simulink model "METI_TRAMI_Thermal_ver01_Jmaab_2018b_Intg"  (R2018b)
settings: Solver=ode8  StartTime=0  StopTime=end_time  FixedStep=sampling_time  RelTol=1e-3
PreLoadFcn:
  | METI_TRAMI_Thermal_ver01_Jmaab_PreLoad;
values from neighbouring files (symbols this model uses):
  degC2K = 273.15    [METI_TRAMI_Thermal_ver01_Jmaab_PreLoad.m]    (also in init_setting_METI.m)
  K2degC = -273.15    [METI_TRAMI_Thermal_ver01_Jmaab_PreLoad.m]    (also in init_setting_METI.m)
undefined symbols (not defined in the file or in its folder): ACC_D_Gain, ACC_I_Gain, ACC_P_Gain, ALT_CNT_ALT_OFF_RPM_HYS_rpm, ALT_CNT_ALT_ON_RPM_HYS_rpm, ALT_CNT_Alter_V_BASE_V, ALT_CNT_Alter_V_Kaisei_V, ALT_CNT_flag_disable_kaisei, ALT_CNT_V_Battely_Kudo_V, ALT_PNT_ALT_GDCurrent_A, ALT_PNT_ALT_GDVolt_V, ALT_PNT_Alter_limit_Current_V_table, ALT_PNT_Alter_limit_Current_V_table_x_rpm, ALT_PNT_Alter_trq_Nm_map, ALT_PNT_Alter_trq_Nm_map_x_rpm, ALT_PNT_Alter_trq_Nm_map_y_Current_A, ALT_PNT_Alter_trq_Nm_map_z_Volt_tgt_V, ALT_PNT_eta_pulley_alt, ALT_PNT_Gain_Alt_v_del, ALT_PNT_ratio_pulley_alt, ALT_PNT_Tau_Alternator_V_tgt_s, ALT_PNT_trq_alter_output_LL_Nm, BK_PNT_Pow_UL, BK_PNT_Tau_brake, Brk_LL, Brk_PGain, Brk_UL, BT_PNT_Lo_Capa_lo_batt_F, BT_PNT_Lo_ocv_SOC_lo_batt_OCV_V_table, BT_PNT_Lo_ocv_SOC_lo_batt_OCV_V_table_x_SOC, BT_PNT_Lo_R_lo_batt_ohm, BT_PNT_Lo_SOC_MAX_lo_batt, BT_PNT_Lo_SOC_MIN_lo_batt, BT_PNT_Lo_SOC_START_lo_batt, BT_PNT_Lo_V_start_ocv, DF_PNT_DF_gear, DF_PNT_DFBlock2DFAir_Heat_Resi_KpW, DF_PNT_DFBlock_Heat_Capa_JpK, DF_PNT_DFBlock_Temp_ini_degC, DF_PNT_DFOil2DFBlock_Heat_Resi_KpW, DF_PNT_DFOil_Heat_Capa_JpK, DF_PNT_DFOil_Temp_ini_degC, DF_PNT_Driveshaft_damper, DF_PNT_Driveshaft_delta_radps_LL, DF_PNT_Driveshaft_delta_radps_UL, DF_PNT_Driveshaft_spring, DF_PNT_eta_DF, DF_PNT_Outtemp_degC, DF_PNT_TMBlock2DFBlock_Heat_Resi_KpW, Driver_Brake_Const1, Driver_Brake_Const3, Driver_Brake_Switch_Const2, Driver_Brk_sh, drivmode_ACC, drivmode_CONST, drivmode_GensokuKaisei, drivmode_GensokuRikko, drivmode_STOP, EL_PNT_R_bodyelec_lo_ohm, ENG_CNT_acc_idlestop ... (+139)
libraries: METI_Lib_vehicle_model x33, simulink x7, AZAPA_Lib_vehicle_model x1
(part 3 of 4)

== system METI_TRAMI_Thermal_ver01_Jmaab_2018b_Intg/Vehicle/PTTH/DTTH_PNT/DTTH_PNT ==
  "TM_CNT_out " : Inport
  "PHI_TM_PNT " : Inport  Port=2
  "T_ENG_TM " : Inport  Port=3
  "T_RD_TM " : Inport  Port=4
  "T_ATM_TM " : Inport  Port=5
  "v_VL_PNT_mps " : Inport  Port=6
  DTTH_PNT : Subsystem  TreatAsAtomicUnit=on  VariantControl=VarObj_METI_Subsys
      settings: AttributesFormatString="<AtomicUnit =  %<TreatAsAtomicUnit>>"
  DTTH_PNT1 : ModelReference  ModelNameDialog=METI_DTTH_PNT  SimulationMode=Normal  VariantControl=VarObj_METI_Mref  ModelReferenceVersion=1.421
  DTTH_PNT2 : ModelReference  ModelNameDialog=TRAMI_DTTH_PNT  SimulationMode=Normal  VariantControl=VarObj_TRAMI_Mref  ModelReferenceVersion=1.396
  " T_TMTH_PNT" : Outport
  " PHI_TM_ENG" : Outport  Port=2
  " PHI_TM_RD" : Outport  Port=3
  " PHI_TM_ATM" : Outport  Port=4
  " TMTH_Info" : Outport  Port=5

== system METI_TRAMI_Thermal_ver01_Jmaab_2018b_Intg/Vehicle/PTTH/ENGTH_PNT/ENGTH ==
  note: エンジンオイル
      | 熱容量
  note: エンジン冷却水
      | 熱容量
  note: エンジンブロック
      | 熱容量
  note: 冷却水からラジエターへ
      | 放熱する熱量
  note: エネルギーの
      | 向きの定義（仮）
      | →→→
  note: エンジン燃焼室からシリンダヘッドへ
      | 放熱する熱量
  note: エンジンからエンジンオイルへ
      | 放熱する熱量
  note: エネルギーの
      | 向きの定義（仮）
      | →→→
  note: エネルギーの
      | 向きの定義（仮）
      | →→→
  note: エネルギーの
      | 向きの定義（仮）
      | →→→
  note: エネルギーの
      | 向きの定義（仮）
      | →→→
  note: エネルギーの
      | 向きの定義（仮）
      | →→→
  note: エネルギーの
      | 向きの定義（仮）
      | →→→
  note: エンジンブロックからT/Mブロックへ
      | 放熱する熱量
  note: シリンダヘッド
      | 熱容量
  note: エネルギーの
      | 向きの定義（仮）
      | →→→
  V_ENG_CNT_WP_V : Inport
  PHI_ENGBlock_W : Inport  Port=2
  PHI_ENG_PNT_Head_W : Inport  Port=3
  PHI_ENG_PNT_Oil_W : Inport  Port=4
  T_ATM_PNT_ENG_K : Inport  Port=5
  PHI_TM_CVTF_Resi_W : Inport  Port=6
  PHI_ENGCoolant_W1 : Inport  Port=7
  Add : Sum
  Coolant_Heat_Capacity : Subsystem
  Cylinder_Head2Coolant_Heat_Resistance : Subsystem
  ENGBlock2Air_Heat_Resistance : Subsystem
  ENGBlock2Coolant_Heat_Resistance : Subsystem
  ENGBlock_Heat_Capacity : Subsystem
  ENGOil2Coolant_Heat_Resistance : Subsystem
  ENGOil_Heat_Capacity : Subsystem
  ENGOil_Heat_Capacity1 : Subsystem
  Water_Pump : Subsystem
  T_ENGTH_PNT_Coolant_K : Outport
  T_ENG_Block_K : Outport  Port=2
  T_ENGTH_PNT_Oil_K : Outport  Port=3
  T_ENGTH_PNT_Head_K : Outport  Port=4
  PHI_ENGTH_PNT_W : Outport  Port=5
  wires:
  PHI_TM_CVTF_Resi_W/1 -> Add/1
  Add/1 -> Coolant_Heat_Capacity/4(PHI_Coolant2_W)  "PHI_ENGCoolant_W"
  ENGOil_Heat_Capacity/1(T_ENGOil2_K) -> ENGOil2Coolant_Heat_Resistance/1(T_ENGOil_Resi2_K)
  ENGOil2Coolant_Heat_Resistance/2(PHI_Coolant_Resi3_W) -> Coolant_Heat_Capacity/3(PHI_Coolant3_W)
  PHI_ENGCoolant_W1/1 -> Add/2
  PHI_ENG_PNT_Head_W/1 -> ENGOil_Heat_Capacity1/1(PHI_Cylinder_Head1_W)
  ENGBlock_Heat_Capacity/3(T_ENGBlock1_K) -> ENGBlock2Coolant_Heat_Resistance/2(T_ENGBlock_Resi1_K)
  ENGBlock_Heat_Capacity/1(T_ENGBlock3_K) -> ENGBlock2Air_Heat_Resistance/1(T_ENGBlock_Resi3_K)
  ENGOil_Heat_Capacity1/1(T_Cylinder_Head1_K) -> T_ENGTH_PNT_Head_K/1  "T_Cylinder_Head0_K"
  Cylinder_Head2Coolant_Heat_Resistance/1(PHI_Coolant_Resi1_W) -> Coolant_Heat_Capacity/2(PHI_Coolant1_W)
  Cylinder_Head2Coolant_Heat_Resistance/2(PHI_Cylinder_Head_Resi2_W) -> ENGOil_Heat_Capacity1/2(PHI_Cylinder_Head2_W)
  Water_Pump/1(Qv_Coolant_m3ps) -> Cylinder_Head2Coolant_Heat_Resistance/2(Qv_Coolant_m3ps)
  ENGBlock_Heat_Capacity/2(T_ENGBlock2_K) -> T_ENG_Block_K/1  "T_ENG_Block_K"
  PHI_ENGBlock_W/1 -> ENGBlock_Heat_Capacity/3(PHI_ENGBlock2_W)
  V_ENG_CNT_WP_V/1 -> Water_Pump/1(ENG_PNT_Voltage_WP_V)
  ENGOil_Heat_Capacity1/2(T_Cylinder_Head2_K) -> Cylinder_Head2Coolant_Heat_Resistance/3(T_Cylinder_Head_Resi2_K)
  ENGBlock2Coolant_Heat_Resistance/1(PHI_Coolant_Resi4_W) -> Coolant_Heat_Capacity/1(PHI_Coolant4_W)
  Coolant_Heat_Capacity/4(T_Coolant3_K) -> ENGOil2Coolant_Heat_Resistance/2(T_Coolant_Resi3_K)
  ENGBlock2Air_Heat_Resistance/1(PHI_ENGBlock_Resi3_W) -> ENGBlock_Heat_Capacity/1(PHI_ENGBlock3_W)
  ENGOil2Coolant_Heat_Resistance/1(PHI_ENGOil_Resi2_W) -> ENGOil_Heat_Capacity/1(PHI_ENGOil2_W)
  Coolant_Heat_Capacity/2(T_Coolant4_K) -> ENGBlock2Coolant_Heat_Resistance/1(T_Coolant_Resi4_K)
  T_ATM_PNT_ENG_K/1 -> ENGBlock2Air_Heat_Resistance/2(T_ENG_Air_Resi1_K)
  ENGBlock2Coolant_Heat_Resistance/2(PHI_ENGBlock_Resi1_W) -> ENGBlock_Heat_Capacity/2(PHI_ENGBlock1_W)
  Coolant_Heat_Capacity/3(T_Coolant2_K) -> T_ENGTH_PNT_Coolant_K/1  "T_ENGTH_PNT_Coolant_K"
  Coolant_Heat_Capacity/1(T_Coolant1_K) -> Cylinder_Head2Coolant_Heat_Resistance/1(T_Coolant_Resi1_K)
  ENGBlock2Air_Heat_Resistance/2(PHI_ENG_Air_Resi1_W) -> PHI_ENGTH_PNT_W/1  "PHI_ENGTH_PNT_W"
  ENGOil_Heat_Capacity/2(T_ENGOil1_K) -> T_ENGTH_PNT_Oil_K/1  "T_ENGOil0_K"
  PHI_ENG_PNT_Oil_W/1 -> ENGOil_Heat_Capacity/2(PHI_ENGOil1_W)

== system METI_TRAMI_Thermal_ver01_Jmaab_2018b_Intg/Vehicle/PTTH/RDTH_PNT/RDTH ==
  note: サーモスタット
  note: エネルギーの
      | 向きの定義（仮）
      | →→→
  note: エネルギーの
      | 向きの定義（仮）
      | →→→
  RD_PNT_Voltage_RDFan_V : Inport
  v_VL_PNT_kmph : Inport  Port=2
  T_ENGTH_PNT_Coolant_K : Inport  Port=3
  T_ATM_PNT_RD_K : Inport  Port=4
  ENGBlock2Coolant_Heat_Resistance : Subsystem
  RDCoolant2Air_Heat_Resistance : Subsystem
  RDCoolant_Heat_Capacity : Subsystem
  RD_Core_Heat_Resi_Calc : Subsystem
  T_RDCoolant_degC : Outport
  PHI_RDTH_PNT_W : Outport  Port=2
  PHI_RD_Air_Resi_W : Outport  Port=3
  tag scope: RD_PNT_RDCore_Heat_Resi_KpW=global
  wires:
  T_ATM_PNT_RD_K/1 -> RDCoolant2Air_Heat_Resistance/1(T_RD_Air_Resi_K)
  RDCoolant_Heat_Capacity/2(T_RDCoolant2_K) -> T_RDCoolant_degC/1, RDCoolant2Air_Heat_Resistance/3(T_RDCoolant_Resi2_K)  "T_RDCoolant_degC"
  RDCoolant_Heat_Capacity/1(T_RDCoolant1_K) -> ENGBlock2Coolant_Heat_Resistance/1(T_RDCoolant_Resi1_K)
  RD_Core_Heat_Resi_Calc/1("RD_PNT_RDCore_Heat_Resi_KpW ") -> [RD_PNT_RDCore_Heat_Resi_KpW], RDCoolant2Air_Heat_Resistance/2("RD_PNT_RDCore_Heat_Resi_KpW ")
  RDCoolant2Air_Heat_Resistance/1(PHI_RD_Air_Resi1_W) -> PHI_RD_Air_Resi_W/1  "PHI_RD_Air_Resi_W"
  T_ENGTH_PNT_Coolant_K/1 -> ENGBlock2Coolant_Heat_Resistance/2(T_Thermostat_Resi1_K)
  ENGBlock2Coolant_Heat_Resistance/2(PHI_Thermostat_Resi1_W) -> PHI_RDTH_PNT_W/1  "PHI_RDTH_PNT_W"
  RDCoolant2Air_Heat_Resistance/2(PHI_RDCoolant_Resi2_W) -> RDCoolant_Heat_Capacity/2(PHI_RDCoolant2_W)
  ENGBlock2Coolant_Heat_Resistance/1(PHI_RDCoolant_Resi1_W) -> RDCoolant_Heat_Capacity/1(PHI_RDCoolant1_W)
  RD_PNT_Voltage_RDFan_V/1 -> RD_Core_Heat_Resi_Calc/1(RD_PNT_Voltage_RDFan_V)
  v_VL_PNT_kmph/1 -> RD_Core_Heat_Resi_Calc/2(v_VL_PNT_kmph)

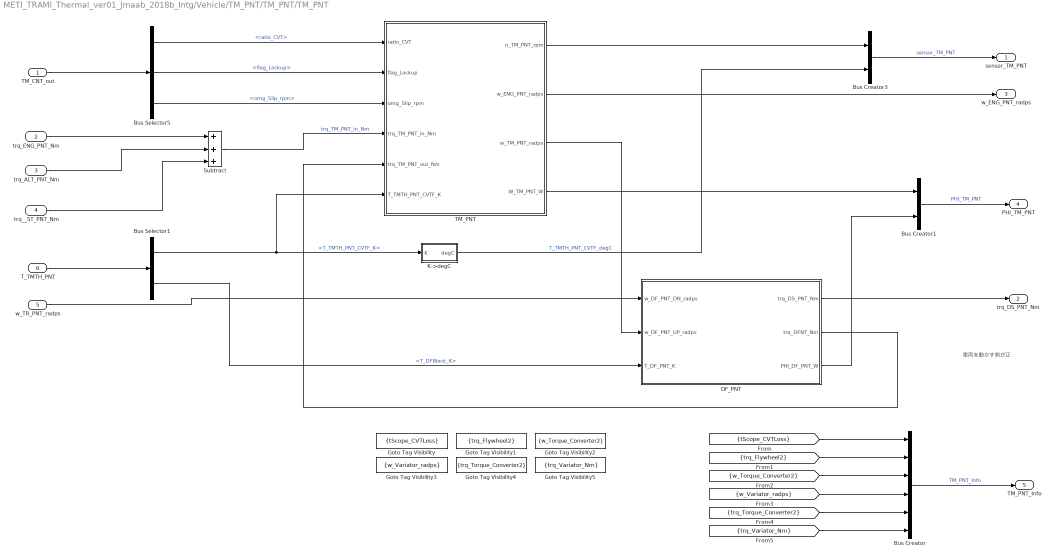
== system METI_TRAMI_Thermal_ver01_Jmaab_2018b_Intg/Vehicle/TM_PNT/TM_PNT/TM_PNT ==
  note: 車両を動かす側が正
  TM_CNT_out : Inport
  trq_ENG_PNT_Nm : Inport  Port=2
  trq_ALT_PNT_Nm : Inport  Port=3
  trq__ST_PNT_Nm : Inport  Port=4
  w_TR_PNT_radps : Inport  Port=5
  T_TMTH_PNT : Inport  Port=6
  Bus Creator : BusCreator  Inputs=6
  Bus Creator1 : BusCreator  Inputs=2
  Bus Creator3 : BusCreator  Inputs=2
  Bus Selector1 : BusSelector  OutputSignals=T_TMTH_PNT_CVTF_K,T_DFBlock_K
  Bus Selector5 : BusSelector  OutputSignals=ratio_CVT,flag_Lockup,omg_Slip_rpm
  DF_PNT : Subsystem
  Goto Tag Visibility : GotoTagVisibility  GotoTag=tScope_CVTLoss
  Goto Tag Visibility1 : GotoTagVisibility  GotoTag=trq_Flywheel2
  Goto Tag Visibility2 : GotoTagVisibility  GotoTag=w_Torque_Converter2
  Goto Tag Visibility3 : GotoTagVisibility  GotoTag=w_Variator_radps
  Goto Tag Visibility4 : GotoTagVisibility  GotoTag=trq_Torque_Converter2
  Goto Tag Visibility5 : GotoTagVisibility  GotoTag=trq_Variator_Nm
  K->degC : Subsystem
  Subtract : Sum  Inputs=3
  TM_PNT : Subsystem
  sensor_TM_PNT : Outport
  trq_DS_PNT_Nm : Outport  Port=2
  w_ENG_PNT_radps : Outport  Port=3
  PHI_TM_PNT : Outport  Port=4
  TM_PNT_Info : Outport  Port=5
  wires:
  DF_PNT/3(PHI_DF_PNT_W) -> Bus Creator1/2
  TM_PNT/4(W_TM_PNT_W) -> Bus Creator1/1
  Bus Selector5/3 -> TM_PNT/3(omg_Slip_rpm)  "<omg_Slip_rpm>"
  trq_ENG_PNT_Nm/1 -> Subtract/1
  Bus Creator3/1 -> sensor_TM_PNT/1  "sensor_TM_PNT"
  trq__ST_PNT_Nm/1 -> Subtract/3
  TM_PNT/2(w_ENG_PNT_radps) -> w_ENG_PNT_radps/1
  K->degC/1(degC) -> Bus Creator3/2  "T_TMTH_PNT_CVTF_degC"
  Bus Selector5/2 -> TM_PNT/2(flag_Lockup)  "<flag_Lockup>"
  Bus Selector1/1 -> TM_PNT/6(T_TMTH_PNT_CVTF_K), K->degC/1(K)  "<T_TMTH_PNT_CVTF_K>"
  DF_PNT/2(trq_DFNT_Nm) -> TM_PNT/5(trq_TM_PNT_out_Nm)
  Bus Selector5/1 -> TM_PNT/1(ratio_CVT)  "<ratio_CVT>"
  trq_ALT_PNT_Nm/1 -> Subtract/2
  TM_PNT/1(n_TM_PNT_rpm) -> Bus Creator3/1
  T_TMTH_PNT/1 -> Bus Selector1/1
  DF_PNT/1(trq_DS_PNT_Nm) -> trq_DS_PNT_Nm/1
  TM_PNT/3(w_TM_PNT_radps) -> DF_PNT/2(w_DF_PNT_UP_radps)
  Bus Creator1/1 -> PHI_TM_PNT/1  "PHI_TM_PNT"
  w_TR_PNT_radps/1 -> DF_PNT/1(w_DF_PNT_DN_radps)
  Subtract/1 -> TM_PNT/4(trq_TM_PNT_in_Nm)  "trq_TM_PNT_in_Nm"
  Bus Selector1/2 -> DF_PNT/3(T_DF_PNT_K)  "<T_DFBlock_K>"
  TM_CNT_out/1 -> Bus Selector5/1
  Bus Creator/1 -> TM_PNT_Info/1  "TM_PNT_Info"
  [tScope_CVTLoss] -> Bus Creator/1
  [trq_Flywheel2] -> Bus Creator/2
  [w_Torque_Converter2] -> Bus Creator/3
  [w_Variator_radps] -> Bus Creator/4
  [trq_Torque_Converter2] -> Bus Creator/5
  [trq_Variator_Nm] -> Bus Creator/6

== system METI_TRAMI_Thermal_ver01_Jmaab_2018b_Intg/Driver/Driver/Driver/Caliculate_Opeining_Accel/FB ==
  delta_v_VL_kmph : Inport
  Acc_D_Gain : Gain  Gain=D_Gain
  Acc_I_Gain : Gain  Gain=I_Gain
  Acc_P_Gain : Gain  Gain=P_Gain
  Acc_P_Gain1 : Gain  Gain=P_Gain
  Derivative : Derivative
  Filter : Subsystem  Commented=through
  Integrator : Integrator
  Memory : Memory
  Product1 : Product
  Saturation2 : Saturate  UpperLimit=1  LowerLimit=0
  Sum : Sum  Inputs=+++
  Terminator : Terminator
  FB_open_accel_per : Outport
  wires:
  Filter/1(Out1) -> Product1/2
  Saturation2/1 -> Acc_P_Gain/1
  Acc_P_Gain/1 -> Product1/1
  Sum/1 -> FB_open_accel_per/1
  Derivative/1 -> Acc_D_Gain/1
  Integrator/1 -> Acc_I_Gain/1
  delta_v_VL_kmph/1 -> Memory/1
  Acc_I_Gain/1 -> Sum/3
  Acc_D_Gain/1 -> Sum/2
  Product1/1 -> Sum/1
  Memory/1 -> Saturation2/1, Filter/1(In1), Acc_P_Gain1/1, Integrator/1, Derivative/1
  Acc_P_Gain1/1 -> Terminator/1

== system METI_TRAMI_Thermal_ver01_Jmaab_2018b_Intg/Driver/Driver/Driver/Caliculate_Opeining_Accel/FF ==
  note: 速度とパワーでF/B出来るようにモデルを用意しておく
      | 切り替えスイッチを作っておく
  v_VL_PNT_kmph : Inport
  target_v_VL_kmph : Inport  Port=2
  pre_n_eng_rpm : Inport  Port=3
  pre_ratio_CVT : Inport  Port=4
  Air_Resistance : Subsystem
  Cal_M_ENG_jiku2 : Subsystem
  Constant1 : Constant  Value=TM_CNT_CVT_ratio_LL
  Constant3 : Constant  Value=tire_r
  Constant4 : Constant  Value=DF_PNT_DF_gear
  Inertial_Resistance : Subsystem
  MinMax : MinMax  Function=max  Inputs=2
  Product8 : Product  Inputs=*/*/  RndMeth=Zero
  Rolling_Resistance : Subsystem
  Sum4 : Sum  Inputs=+++
  Terminator : Terminator
  Transfer Fcn : TransferFcn  Denominator=[TM_PNT_Tau_CVT_ratio_s 1]
  kmph2mps : Gain  Gain=kmph2mps
  kmph2mps1 : Gain  Gain=kmph2mps
  FF_open_accel_per : Outport
  wires:
  kmph2mps/1 -> Inertial_Resistance/1(V_tgt), Rolling_Resistance/1(V_tgt), Air_Resistance/1(V_tgt)
  target_v_VL_kmph/1 -> kmph2mps/1
  Sum4/1 -> Product8/1
  Constant4/1 -> Product8/2
  Constant3/1 -> Product8/3
  Air_Resistance/1(F_air_resi) -> Sum4/2
  Rolling_Resistance/1(F_rollresi) -> Sum4/3
  Inertial_Resistance/1(F_Inertia) -> Sum4/1
  pre_ratio_CVT/1 -> Transfer Fcn/1
  Constant1/1 -> MinMax/2
  MinMax/1 -> Product8/4
  Transfer Fcn/1 -> MinMax/1
  v_VL_PNT_kmph/1 -> kmph2mps1/1
  kmph2mps1/1 -> Terminator/1
  Cal_M_ENG_jiku2/1(FF_open_accel_per) -> FF_open_accel_per/1
  Product8/1 -> Cal_M_ENG_jiku2/1(FF_trq_accel_Nm)  "FF_trq_accel_Nm"
  pre_n_eng_rpm/1 -> Cal_M_ENG_jiku2/2(pre_n_eng_rpm)

== system METI_TRAMI_Thermal_ver01_Jmaab_2018b_Intg/Driver/Driver_TRAMI/Driver2/Caliculate_Opeining_Accel/FB ==
  delta_v_VL_kmph : Inport
  Acc_D_Gain : Gain  Gain=D_Gain
  Acc_I_Gain : Gain  Gain=I_Gain
  Acc_P_Gain : Gain  Gain=P_Gain
  Acc_P_Gain1 : Gain  Gain=P_Gain
  Derivative : Derivative
  Filter : Subsystem  Commented=through
  Integrator : Integrator
  Memory : Memory
  Product1 : Product
  Saturation2 : Saturate  UpperLimit=1  LowerLimit=0
  Sum : Sum  Inputs=+++
  Terminator : Terminator
  FB_open_accel_per : Outport
  wires:
  Filter/1(Out1) -> Product1/2
  Saturation2/1 -> Acc_P_Gain/1
  Acc_P_Gain/1 -> Product1/1
  Sum/1 -> FB_open_accel_per/1
  Derivative/1 -> Acc_D_Gain/1
  Integrator/1 -> Acc_I_Gain/1
  delta_v_VL_kmph/1 -> Memory/1
  Acc_I_Gain/1 -> Sum/3
  Acc_D_Gain/1 -> Sum/2
  Product1/1 -> Sum/1
  Memory/1 -> Saturation2/1, Filter/1(In1), Acc_P_Gain1/1, Integrator/1, Derivative/1
  Acc_P_Gain1/1 -> Terminator/1

== system METI_TRAMI_Thermal_ver01_Jmaab_2018b_Intg/Driver/Driver_TRAMI/Driver2/Caliculate_Opeining_Accel/FF ==
  note: 速度とパワーでF/B出来るようにモデルを用意しておく
      | 切り替えスイッチを作っておく
  v_VL_PNT_kmph : Inport
  target_v_VL_kmph : Inport  Port=2
  pre_n_eng_rpm : Inport  Port=3
  pre_ratio_DCT : Inport  Port=4
  Air_Resistance : Subsystem
  Cal_M_ENG_jiku2 : Subsystem
  Constant : Constant  Value=0.1
  Constant3 : Constant  Value=tire_r
  Constant4 : Constant  Value=TM_PNT_FD_gear
  Inertial_Resistance : Subsystem
  MinMax : MinMax  Function=max  Inputs=2
  Product8 : Product  Inputs=*/*/  RndMeth=Zero
  Rolling_Resistance : Subsystem
  Sum4 : Sum  Inputs=+++
  Terminator : Terminator
  kmph2mps : Gain  Gain=kmph2mps
  kmph2mps1 : Gain  Gain=kmph2mps
  FF_open_accel_per : Outport
  wires:
  kmph2mps/1 -> Inertial_Resistance/1(V_tgt), Rolling_Resistance/1(V_tgt), Air_Resistance/1(V_tgt)
  target_v_VL_kmph/1 -> kmph2mps/1
  Sum4/1 -> Product8/1
  Constant4/1 -> Product8/2
  Constant3/1 -> Product8/3
  Air_Resistance/1(F_air_resi) -> Sum4/2
  Rolling_Resistance/1(F_rollresi) -> Sum4/3
  Inertial_Resistance/1(F_Inertia) -> Sum4/1
  pre_ratio_DCT/1 -> MinMax/2
  v_VL_PNT_kmph/1 -> kmph2mps1/1
  kmph2mps1/1 -> Terminator/1
  Cal_M_ENG_jiku2/1(FF_open_accel_per) -> FF_open_accel_per/1
  Product8/1 -> Cal_M_ENG_jiku2/1(FF_trq_accel_Nm)  "FF_trq_accel_Nm"
  pre_n_eng_rpm/1 -> Cal_M_ENG_jiku2/2(pre_n_eng_rpm)
  Constant/1 -> MinMax/1
  MinMax/1 -> Product8/4

== system METI_TRAMI_Thermal_ver01_Jmaab_2018b_Intg/Vehicle/ALT_PNT/Subsystem/I_alt_cal/Cal_I_alt_P_control ==
  note: 目標電圧よりもオルタネータ電圧が低い場合電流をPI制御で出力
      | 高い場合は、電流を0とする
  V_delt_tgt : Inport
  Gain : Gain  Gain=ALT_PNT_Gain_Alt_v_del
  Transfer Fcn : TransferFcn  Denominator=[ALT_PNT_Tau_Alternator_V_tgt_s 1]
  I_alt_base : Outport
  wires:
  Gain/1 -> I_alt_base/1
  V_delt_tgt/1 -> Transfer Fcn/1
  Transfer Fcn/1 -> Gain/1

== system METI_TRAMI_Thermal_ver01_Jmaab_2018b_Intg/Vehicle/ALT_PNT/Subsystem/I_alt_cal/Cal_I_alt_base ==
  note: 目標電圧よりもオルタネータ電圧が低い場合電流をPI制御で出力
      | 高い場合は、電流を0とする
  V_delt_tgt : Inport
  Constant : Constant  Value=0
  Gain : Gain  Gain=1/BT_PNT_Lo_R_lo_batt_ohm
  MinMax : MinMax  Function=max  Inputs=2
  Switch : Switch  Criteria=u2 > Threshold
  Transfer Fcn : TransferFcn  Denominator=[ALT_PNT_Tau_Alternator_V_tgt_s 1]
  I_alt_base : Outport
  wires:
  MinMax/1 -> I_alt_base/1
  Gain/1 -> Switch/1
  V_delt_tgt/1 -> Transfer Fcn/1
  Constant/1 -> MinMax/2, Switch/3
  Switch/1 -> MinMax/1
  Transfer Fcn/1 -> Switch/2, Gain/1

== system METI_TRAMI_Thermal_ver01_Jmaab_2018b_Intg/Vehicle/CNT/ENG_CNT/ENG_Cntrl/Caliculate_Idle_Speed ==
  note: 補機負荷やNDの時の負荷によるアイドル安定化処理を入れる
      | パワーデマンドで締結
  note: ○目標回転数に対するP制御
  note: 目標アイドル回転数
  per_throttle_base : Inport
  n_eng_rpm : Inport  Port=2
  flag_Lockup : Inport  Port=3
  flag_IdleStop : Inport  Port=4
  T_ENGTH_PNT_Coolant_dC : Inport  Port=5
  Subsystem : Subsystem
  Subsystem1 : Subsystem
  Subtract : Sum  Inputs=+-
  Tw2ENG_CNT_IdleSpeed : Lookup_n-D  NumberOfTableDimensions=1  BreakpointsForDimension1=T_ENGCoodant_T_ENGCoodant  Table=ENG_CNT_IdleSpeed  InternalRulePriority=Speed  RndMeth=Simplest  InputSameDT=on
  per_isc_[%] : Outport
  IdleSpeed_Target : Outport  Port=2
  tag scope: ENG_CNT_IdleSpeed=global
  wires:
  Tw2ENG_CNT_IdleSpeed/1 -> Subtract/1, Subsystem1/1(omg_tgt_idle), IdleSpeed_Target/1, [ENG_CNT_IdleSpeed]  "IdleSpeed_Target"
  T_ENGTH_PNT_Coolant_dC/1 -> Tw2ENG_CNT_IdleSpeed/1
  Subsystem/1(per_isc_[%]) -> per_isc_[%]/1
  flag_IdleStop/1 -> Subsystem1/5(flag_IdleStop)
  Subsystem1/1(flag_idle_fb) -> Subsystem/2(flag_idle_fb)
  flag_Lockup/1 -> Subsystem1/4(flag_Lockup)
  per_throttle_base/1 -> Subsystem1/3(per_throttle_base)
  Subtract/1 -> Subsystem/1(del_omg_engine)
  n_eng_rpm/1 -> Subtract/2, Subsystem1/2(n_eng_rpm)

== system METI_TRAMI_Thermal_ver01_Jmaab_2018b_Intg/Vehicle/CNT/ENG_CNT/ENG_Cntrl/Injection_Control ==
  T_ENGTH_PNT_Coolant_dC : Inport
  Tw2KFuel : Lookup_n-D  NumberOfTableDimensions=1  BreakpointsForDimension1=T_ENGCoodant  Table=K_Fuel  RndMeth=Simplest  InputSameDT=on
  K_Fuel : Outport
  wires:
  T_ENGTH_PNT_Coolant_dC/1 -> Tw2KFuel/1
  Tw2KFuel/1 -> K_Fuel/1  "K_Fuel"

== system METI_TRAMI_Thermal_ver01_Jmaab_2018b_Intg/Vehicle/CNT/ENG_CNT/ENG_Cntrl/K->degC7 ==
  K : Inport
  Constant2 : Constant  Value=K2degC
  Sum : Sum  Inputs=++|
  degC : Outport
  wires:
  K/1 -> Sum/2
  Constant2/1 -> Sum/1
  Sum/1 -> degC/1

== system METI_TRAMI_Thermal_ver01_Jmaab_2018b_Intg/Vehicle/CNT/ENG_CNT/ENG_Cntrl/RD_Fan_Control ==
  T_ENGTH_PNT_Coolant_dC : Inport
  1-D Lookup Table1 : Lookup_n-D  NumberOfTableDimensions=1  BreakpointsForDimension1=ENG_CNT_V_RDFan_x_T_Coolant  BeginIndexSearchUsingPreviousIndexResult=on  Table=ENG_CNT_V_RDFan_V  InternalRulePriority=Speed  RndMeth=Simplest  InputSameDT=on
  V_RDTH_PNT_Fan_V : Outport
  wires:
  1-D Lookup Table1/1 -> V_RDTH_PNT_Fan_V/1
  T_ENGTH_PNT_Coolant_dC/1 -> 1-D Lookup Table1/1

== system METI_TRAMI_Thermal_ver01_Jmaab_2018b_Intg/Vehicle/CNT/ENG_CNT/ENG_Cntrl/Set_Fuel_Cut ==
  note: ○減速時のフューエルカット条件
      | 　・停車中でない
      | 　・回転数がある回転数以上
      | 　・アクセル開度がOFF
  v_vehicle : Inport
  n_eng_rpm : Inport  Port=2
  per_throttle_base : Inport  Port=3
  Constant1 : Constant  Value=ENG_CNT_V_vhicle_fuelcut_kmph
  Constant4 : Constant  Value=ENG_CNT_omg_eng_fuelcut_rpm
  Constant6 : Constant  Value=ENG_CNT_per_throttle_fuelcut
  Logical Operator : Logic  Inputs=3  AllPortsSameDT=off  OutDataTypeStr=boolean
  Relational Operator1 : RelationalOperator  Operator=<=  OutDataTypeStr=boolean  RndMeth=Nearest
  Relational Operator2 : RelationalOperator  OutDataTypeStr=boolean  RndMeth=Nearest
  Relational Operator3 : RelationalOperator  OutDataTypeStr=boolean  RndMeth=Nearest
  flag_fuelcut : Outport
  wires:
  Constant4/1 -> Relational Operator2/2
  Relational Operator3/1 -> Logical Operator/1
  v_vehicle/1 -> Relational Operator3/1
  Constant1/1 -> Relational Operator3/2
  Logical Operator/1 -> flag_fuelcut/1
  Relational Operator2/1 -> Logical Operator/2
  Relational Operator1/1 -> Logical Operator/3
  Constant6/1 -> Relational Operator1/2
  per_throttle_base/1 -> Relational Operator1/1
  n_eng_rpm/1 -> Relational Operator2/1

== system METI_TRAMI_Thermal_ver01_Jmaab_2018b_Intg/Vehicle/CNT/ENG_CNT/ENG_Cntrl/Set_Idle_Stop ==
  note: ○アイドリングストップ制御
      | 　停車時＋ブレーキを踏んでいるとき、アイドリングストップ
  open_accel_per : Inport
  v_vehicle : Inport  Port=2
  per_brake : Inport  Port=3
  T_ENGTH_PNT_Coolant_dC : Inport  Port=4
  Constant : Constant  Value=ENG_CNT_V_car_idlestop_kmph
  Constant1 : Constant  Value=ENG_CNT_brak_idlestop
  Constant2 : Constant  Value=ENG_CNT_flag_idle_stop_exe
  Constant3 : Constant  Value=ENG_CNT_acc_idlestop
  Logical Operator : Logic  Inputs=5  AllPortsSameDT=off  OutDataTypeStr=boolean
  Relational Operator : RelationalOperator  Operator=<  OutDataTypeStr=boolean  RndMeth=Nearest
  Relational Operator1 : RelationalOperator  OutDataTypeStr=boolean  RndMeth=Nearest
  Relational Operator2 : RelationalOperator  Operator=<  OutDataTypeStr=boolean  RndMeth=Nearest
  Relay : Relay  OnSwitchValue=ENG_CNT_IdleStop_flag_const  OffSwitchValue=ENG_CNT_IdleStop_flag_const-5
  flag_IdleStop : Outport
  wires:
  Relational Operator2/1 -> Logical Operator/5
  Constant3/1 -> Relational Operator2/2
  open_accel_per/1 -> Relational Operator2/1
  Relay/1 -> Logical Operator/4
  T_ENGTH_PNT_Coolant_dC/1 -> Relay/1
  Constant2/1 -> Logical Operator/1
  Relational Operator1/1 -> Logical Operator/3
  Constant1/1 -> Relational Operator1/2
  Constant/1 -> Relational Operator/2
  per_brake/1 -> Relational Operator1/1
  v_vehicle/1 -> Relational Operator/1
  Logical Operator/1 -> flag_IdleStop/1
  Relational Operator/1 -> Logical Operator/2

== system METI_TRAMI_Thermal_ver01_Jmaab_2018b_Intg/Vehicle/CNT/ENG_CNT/ENG_Cntrl/Starter ==
  note: アイドリングフラグがON→OFFに切り替わり時スターターON開始.ある時間を超えたらOFF
  note: スタータ開始時間から
      | ある時間超えたらOFF
  note: スタータ開始時間
  note: アイドリングフラグがON→OFFに
      | 切り替わり時スターターON開始
  note: 時間リセット
  note: サンプリング時間
  flag_idlestop : Inport
  n_eng_rpm : Inport  Port=2
  Constant2 : Constant  Value=ENG_CNT_Starter_timer_Const_s
  Constant4 : Constant  Value=sampling_time
  Constant5 : Constant  Value=0
  Constant6 : Constant  Value=OFF
  Constant7 : Constant  Value=ON
  IdleSpeed : Constant  Value=ENG_CNT_IdleSpeed_Const/2
  Logical Operator : Logic  Inputs=3  AllPortsSameDT=off  OutDataTypeStr=boolean
  Logical Operator1 : Logic  Operator=NOT  AllPortsSameDT=off  OutDataTypeStr=boolean
  Memory : Memory  InitialCondition=1000
  Memory1 : Memory  InheritSampleTime=on
  Relational Operator1 : RelationalOperator  Operator=<=  OutDataTypeStr=boolean  RndMeth=Nearest
  Relational Operator2 : RelationalOperator  Operator=<  OutDataTypeStr=boolean  RndMeth=Nearest
  Sum5 : Sum  Inputs=|++
  Switch3 : Switch  Criteria=u2 > Threshold  Threshold=0.5
  Switch4 : Switch  Criteria=u2 > Threshold  Threshold=0.5
  flag_ON_Starter : Outport
  wires:
  Relational Operator2/1 -> Logical Operator/3
  IdleSpeed/1 -> Relational Operator2/2
  n_eng_rpm/1 -> Relational Operator2/1
  Constant6/1 -> Switch4/3
  Constant7/1 -> Switch4/1
  Relational Operator1/1 -> Switch4/2
  Constant2/1 -> Relational Operator1/2
  Logical Operator/1 -> Switch3/2
  flag_idlestop/1 -> Logical Operator1/1, Memory1/1
  Logical Operator1/1 -> Logical Operator/1
  Memory1/1 -> Logical Operator/2
  Switch3/1 -> Memory/1, Relational Operator1/1
  Sum5/1 -> Switch3/3
  Constant5/1 -> Switch3/1
  Constant4/1 -> Sum5/1
  Memory/1 -> Sum5/2
  Switch4/1 -> flag_ON_Starter/1

== system METI_TRAMI_Thermal_ver01_Jmaab_2018b_Intg/Vehicle/CNT/ENG_CNT/ENG_Cntrl/Water_Pump_Control ==
  T_ENGTH_PNT_Coolant_dC : Inport
  1-D Lookup Table1 : Lookup_n-D  NumberOfTableDimensions=1  BreakpointsForDimension1=ENG_CNT_V_Water_Pump_x_T_Coolant  BeginIndexSearchUsingPreviousIndexResult=on  Table=ENG_CNT_V_Water_Pump_V  InternalRulePriority=Speed  RndMeth=Simplest  InputSameDT=on
  V_ENG_PNT_WP_V : Outport
  wires:
  1-D Lookup Table1/1 -> V_ENG_PNT_WP_V/1
  T_ENGTH_PNT_Coolant_dC/1 -> 1-D Lookup Table1/1

== system METI_TRAMI_Thermal_ver01_Jmaab_2018b_Intg/Vehicle/CNT/TM_CNT/TM_CNT/TM_CNT ==
  "sensor_TM_PNT " : Inport  SampleTime=0.01
      settings: AttributesFormatString=<SampleTime = %<SampleTime>>
  TM_CNT_CAN_Rx : Inport  Port=2  SampleTime=0.01
      settings: AttributesFormatString=<SampleTime = %<SampleTime>>
  Bus Creator : BusCreator  Inputs=2
  Bus Creator1 : BusCreator  Inputs=4
  Bus Creator2 : BusCreator  Inputs=2
  Bus Selector1 : BusSelector  OutputSignals=v_VL_PNT_kmph,T_ENGTH_PNT_Coolant_degC,open_throttle_per
  Bus Selector2 : BusSelector  OutputSignals=n_TM_PNT_rpm,T_TMTH_PNT_CVTF_degC
  Goto Tag Visibility : GotoTagVisibility  GotoTag=tScope_Luckup
  Goto Tag Visibility1 : GotoTagVisibility  GotoTag=tScope_CVTratio
  TM_Ctrl : Subsystem
  TM_CNT_out : Outport
  TM_CNT_CAN_Tx : Outport  Port=2
  TM_CNT_Info : Outport  Port=3
  wires:
  Bus Selector2/2 -> TM_Ctrl/3(T_TMTH_PNT_CVTF_degC)  "<T_TMTH_PNT_CVTF_degC>"
  Bus Selector1/3 -> TM_Ctrl/5(open_throttle_per)  "<open_throttle_per>"
  TM_Ctrl/2(omg_Slip_rpm) -> Bus Creator1/2, Bus Creator/2
  Bus Selector1/1 -> TM_Ctrl/1(v_VL_PNT_kmph)  "<v_VL_PNT_kmph>"
  [tScope_Luckup] -> Bus Creator2/1
  TM_Ctrl/1(flag_Lockup) -> Bus Creator1/1, Bus Creator/1
  [tScope_CVTratio] -> Bus Creator2/2
  Bus Selector2/1 -> TM_Ctrl/2(n_TM_PNT_rpm)  "<n_TM_PNT_rpm>"
  TM_Ctrl/3(ratio_CVT) -> Bus Creator1/3
  Bus Creator1/1 -> TM_CNT_out/1  "TM_CNT_out"
  "sensor_TM_PNT "/1 -> Bus Selector2/1
  TM_Ctrl/4(R_CVTF_warmer_tgt_KpW) -> Bus Creator1/4
  Bus Selector1/2 -> TM_Ctrl/4(T_ENGTH_PNT_Coolant_degC)  "<T_ENGTH_PNT_Coolant_degC>"
  Bus Creator2/1 -> TM_CNT_Info/1  "TM_CNT_Info"
  TM_CNT_CAN_Rx/1 -> Bus Selector1/1
  Bus Creator/1 -> TM_CNT_CAN_Tx/1  "TM_CNT_CAN_Tx"

== system METI_TRAMI_Thermal_ver01_Jmaab_2018b_Intg/Vehicle/ENG_PNT/ENG_Plant/Cal_FuelComsunption/Not_cal1 ==
  In1 : Inport
  Constant : Constant  Value=0
  Constant1 : Constant
  Switch : Switch  Criteria=u2 > Threshold  Threshold=0.5
  Out1 : Outport
  wires:
  Constant1/1 -> Switch/3
  Constant/1 -> Switch/1
  Switch/1 -> Out1/1
  In1/1 -> Switch/2

== system METI_TRAMI_Thermal_ver01_Jmaab_2018b_Intg/Vehicle/ENG_PNT/ENG_Plant/Cal_FuelComsunption/Not_cal2 ==
  In1 : Inport
  Constant : Constant  Value=0
  Constant1 : Constant
  Switch : Switch  Criteria=u2 > Threshold  Threshold=0.5
  Out1 : Outport
  wires:
  In1/1 -> Switch/2
  Switch/1 -> Out1/1
  Constant/1 -> Switch/1
  Constant1/1 -> Switch/3

== system METI_TRAMI_Thermal_ver01_Jmaab_2018b_Intg/Vehicle/ENG_PNT/ENG_Plant/Cal_trq_ENG_jiku/Not_cal ==
  In1 : Inport
  Constant : Constant  Value=0
  Constant1 : Constant
  Switch : Switch  Criteria=u2 > Threshold  Threshold=0.5
  Out1 : Outport
  wires:
  In1/1 -> Switch/2
  Switch/1 -> Out1/1
  Constant/1 -> Switch/1
  Constant1/1 -> Switch/3

== system METI_TRAMI_Thermal_ver01_Jmaab_2018b_Intg/Vehicle/ENG_PNT/ENG_Plant/Cal_trq_ENG_jiku/Not_cal1 ==
  In1 : Inport
  Constant : Constant  Value=0
  Constant1 : Constant
  Switch : Switch  Criteria=u2 > Threshold  Threshold=0.5
  Out1 : Outport
  wires:
  Constant1/1 -> Switch/3
  Constant/1 -> Switch/1
  Switch/1 -> Out1/1
  In1/1 -> Switch/2

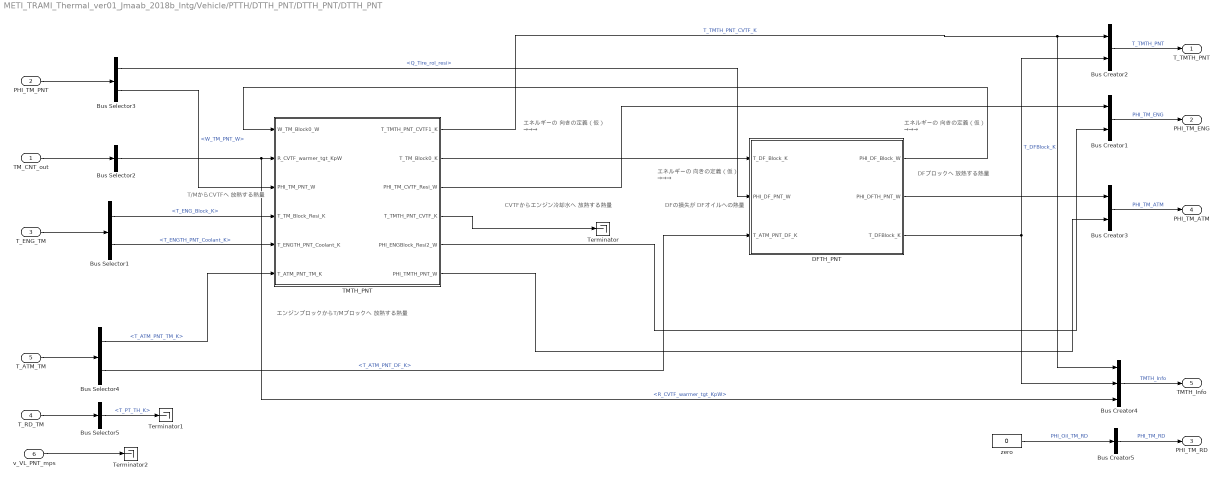
== system METI_TRAMI_Thermal_ver01_Jmaab_2018b_Intg/Vehicle/PTTH/DTTH_PNT/DTTH_PNT/DTTH_PNT ==
  note: DFブロックへ
      | 放熱する熱量
  note: CVTFからエンジン冷却水へ
      | 放熱する熱量
  note: エンジンブロックからT/Mブロックへ
      | 放熱する熱量
  note: エネルギーの
      | 向きの定義（仮）
      | →→→
  note: エネルギーの
      | 向きの定義（仮）
      | →→→
  note: エネルギーの
      | 向きの定義（仮）
      | →→→
  note: T/MからCVTFへ
      | 放熱する熱量
  note: DFの損失が
      | DFオイルへの熱量
  TM_CNT_out : Inport
  PHI_TM_PNT : Inport  Port=2
  T_ENG_TM : Inport  Port=3
  T_RD_TM : Inport  Port=4
  T_ATM_TM : Inport  Port=5
  v_VL_PNT_mps : Inport  Port=6
  Bus Creator1 : BusCreator  Inputs=2
  Bus Creator2 : BusCreator  Inputs=2
  Bus Creator3 : BusCreator  Inputs=2
  Bus Creator4 : BusCreator  Inputs=3
  Bus Creator5 : BusCreator  Inputs=1
  Bus Selector1 : BusSelector  OutputSignals=T_ENG_Block_K,T_ENGTH_PNT_Coolant_K
  Bus Selector2 : BusSelector  OutputSignals=R_CVTF_warmer_tgt_KpW
  Bus Selector3 : BusSelector  OutputSignals=Q_Tire_rol_resi,W_TM_PNT_W
  Bus Selector4 : BusSelector  OutputSignals=T_ATM_PNT_TM_K,T_ATM_PNT_DF_K
  Bus Selector5 : BusSelector  OutputSignals=T_PT_TH_K
  DFTH_PNT : Subsystem
      mask Display: image(imread('picture\回転変換.png'))
  TMTH_PNT : Subsystem
      mask Display: image(imread('picture\image\トランスミッション02.jpg'))
  Terminator : Terminator
  Terminator1 : Terminator
  Terminator2 : Terminator
  zero : Constant  Value=0
  T_TMTH_PNT : Outport
  PHI_TM_ENG : Outport  Port=2
  PHI_TM_RD : Outport  Port=3
  PHI_TM_ATM : Outport  Port=4
  TMTH_Info : Outport  Port=5
  wires:
  DFTH_PNT/2(PHI_DFTH_PNT_W) -> Bus Creator3/1
  Bus Selector4/2 -> DFTH_PNT/3(T_ATM_PNT_DF_K)  "<T_ATM_PNT_DF_K>"
  TMTH_PNT/4(T_TMTH_PNT_CVTF_K) -> Terminator/1
  TMTH_PNT/2(T_TM_Block0_K) -> DFTH_PNT/1(T_DF_Block_K)
  DFTH_PNT/1(PHI_DF_Block_W) -> TMTH_PNT/1(W_TM_Block0_W)
  TMTH_PNT/6(PHI_TMTH_PNT_W) -> Bus Creator3/2
  TMTH_PNT/5(PHI_ENGBlock_Resi2_W) -> Bus Creator1/2
  TMTH_PNT/3(PHI_TM_CVTF_Resi_W) -> Bus Creator1/1
  T_ENG_TM/1 -> Bus Selector1/1
  Bus Selector1/1 -> TMTH_PNT/4(T_TM_Block_Resi_K)  "<T_ENG_Block_K>"
  Bus Selector1/2 -> TMTH_PNT/5(T_ENGTH_PNT_Coolant_K)  "<T_ENGTH_PNT_Coolant_K>"
  TMTH_PNT/1(T_TMTH_PNT_CVTF1_K) -> Bus Creator4/1, Bus Creator2/1  "T_TMTH_PNT_CVTF_K"
  DFTH_PNT/3(T_DFBlock_K) -> Bus Creator4/2, Bus Creator2/2  "T_DFBlock_K"
  Bus Creator2/1 -> T_TMTH_PNT/1  "T_TMTH_PNT"
  Bus Creator1/1 -> PHI_TM_ENG/1  "PHI_TM_ENG"
  Bus Creator3/1 -> PHI_TM_ATM/1  "PHI_TM_ATM"
  Bus Creator4/1 -> TMTH_Info/1  "TMTH_Info"
  PHI_TM_PNT/1 -> Bus Selector3/1
  Bus Selector3/2 -> TMTH_PNT/3(PHI_TM_PNT_W)  "<W_TM_PNT_W>"
  Bus Selector3/1 -> DFTH_PNT/2(PHI_DF_PNT_W)  "<Q_Tire_rol_resi>"
  TM_CNT_out/1 -> Bus Selector2/1
  Bus Selector2/1 -> Bus Creator4/3, TMTH_PNT/2(R_CVTF_warmer_tgt_KpW)  "<R_CVTF_warmer_tgt_KpW>"
  T_ATM_TM/1 -> Bus Selector4/1
  Bus Selector4/1 -> TMTH_PNT/6(T_ATM_PNT_TM_K)  "<T_ATM_PNT_TM_K>"
  Bus Creator5/1 -> PHI_TM_RD/1  "PHI_TM_RD"
  zero/1 -> Bus Creator5/1  "PHI_Oil_TM_RD"
  T_RD_TM/1 -> Bus Selector5/1
  Bus Selector5/1 -> Terminator1/1  "<T_PT_TH_K>"
  v_VL_PNT_mps/1 -> Terminator2/1

== system METI_TRAMI_Thermal_ver01_Jmaab_2018b_Intg/Vehicle/PTTH/ENGTH_PNT/ENGTH/Coolant_Heat_Capacity ==
  PHI_Coolant4_W : Inport
  PHI_Coolant1_W : Inport  Port=2
  PHI_Coolant3_W : Inport  Port=3
  PHI_Coolant2_W : Inport  Port=4
  Add : Sum  Inputs=++++
  Add1 : Sum
  Constant : Constant  Value=ENG_PNT_Coolant_Heat_Capa_JpK
  Constant1 : Constant  Value=ENG_PNT_Coolant_Temp_ini_degC
  Divide : Product  Inputs=/*
  Integrator : Integrator
  degC->K : Subsystem
  T_Coolant1_K : Outport
  T_Coolant4_K : Outport  Port=2
  T_Coolant2_K : Outport  Port=3
  T_Coolant3_K : Outport  Port=4
  wires:
  PHI_Coolant2_W/1 -> Add/4
  PHI_Coolant1_W/1 -> Add/1
  Constant/1 -> Divide/1
  Add/1 -> Divide/2
  Divide/1 -> Integrator/1
  Integrator/1 -> Add1/2
  Add1/1 -> T_Coolant3_K/1, T_Coolant2_K/1, T_Coolant4_K/1, T_Coolant1_K/1
  PHI_Coolant3_W/1 -> Add/2
  PHI_Coolant4_W/1 -> Add/3
  degC->K/1(K) -> Add1/1
  Constant1/1 -> degC->K/1(degC)

== system METI_TRAMI_Thermal_ver01_Jmaab_2018b_Intg/Vehicle/PTTH/ENGTH_PNT/ENGTH/Cylinder_Head2Coolant_Heat_Resistance ==
  T_Coolant_Resi1_K : Inport
  Qv_Coolant_m3ps : Inport  Port=2
  T_Cylinder_Head_Resi2_K : Inport  Port=3
  1-D Lookup Table : Lookup_n-D  NumberOfTableDimensions=1  BreakpointsForDimension1=ENG_PNT_Cylinder_Head2Coolant_Heat_Resi_x_qv_Coolant  Table=ENG_PNT_Cylinder_Head2Coolant_Heat_Resi_KpW  InternalRulePriority=Speed  RndMeth=Simplest  InputSameDT=on
  Add : Sum  Inputs=+-
  Divide : Product  Inputs=*/
  Gain : Gain  Gain=-1
  Gain1 : Gain
  PHI_Coolant_Resi1_W : Outport
  PHI_Cylinder_Head_Resi2_W : Outport  Port=2
  wires:
  T_Cylinder_Head_Resi2_K/1 -> Add/1
  T_Coolant_Resi1_K/1 -> Add/2
  1-D Lookup Table/1 -> Divide/2
  Add/1 -> Divide/1
  Divide/1 -> Gain/1, Gain1/1
  Gain/1 -> PHI_Cylinder_Head_Resi2_W/1
  Gain1/1 -> PHI_Coolant_Resi1_W/1
  Qv_Coolant_m3ps/1 -> 1-D Lookup Table/1

== system METI_TRAMI_Thermal_ver01_Jmaab_2018b_Intg/Vehicle/PTTH/ENGTH_PNT/ENGTH/ENGBlock2Air_Heat_Resistance ==
  T_ENGBlock_Resi3_K : Inport
  T_ENG_Air_Resi1_K : Inport  Port=2
  Add : Sum  Inputs=+-
  Constant : Constant  Value=ENG_PNT_ENGBlock2ENGAir_Heat_Resi_KpW
  Divide : Product  Inputs=*/
  Gain : Gain  Gain=-1
  Gain1 : Gain
  PHI_ENGBlock_Resi3_W : Outport
  PHI_ENG_Air_Resi1_W : Outport  Port=2
  wires:
  Constant/1 -> Divide/2
  Add/1 -> Divide/1
  Divide/1 -> Gain1/1, Gain/1
  Gain/1 -> PHI_ENGBlock_Resi3_W/1
  T_ENGBlock_Resi3_K/1 -> Add/1
  T_ENG_Air_Resi1_K/1 -> Add/2
  Gain1/1 -> PHI_ENG_Air_Resi1_W/1

== system METI_TRAMI_Thermal_ver01_Jmaab_2018b_Intg/Vehicle/PTTH/ENGTH_PNT/ENGTH/ENGBlock2Coolant_Heat_Resistance ==
  T_Coolant_Resi4_K : Inport
  T_ENGBlock_Resi1_K : Inport  Port=2
  Add : Sum  Inputs=+-
  Constant : Constant  Value=ENG_PNT_Coolant2ENGBlock_Heat_Resi_KpW
  Divide : Product  Inputs=*/
  Gain : Gain  Gain=-1
  Gain1 : Gain
  PHI_Coolant_Resi4_W : Outport
  PHI_ENGBlock_Resi1_W : Outport  Port=2
  wires:
  Constant/1 -> Divide/2
  Add/1 -> Divide/1
  Divide/1 -> Gain1/1, Gain/1
  Gain/1 -> PHI_Coolant_Resi4_W/1
  T_Coolant_Resi4_K/1 -> Add/1
  T_ENGBlock_Resi1_K/1 -> Add/2
  Gain1/1 -> PHI_ENGBlock_Resi1_W/1

== system METI_TRAMI_Thermal_ver01_Jmaab_2018b_Intg/Vehicle/PTTH/ENGTH_PNT/ENGTH/ENGBlock_Heat_Capacity ==
  PHI_ENGBlock3_W : Inport
  PHI_ENGBlock1_W : Inport  Port=2
  PHI_ENGBlock2_W : Inport  Port=3
  Add : Sum  Inputs=+++
  Add1 : Sum
  Constant : Constant  Value=ENG_PNT_ENGBlock_Heat_Capa_JpK
  Constant1 : Constant  Value=ENG_PNT_ENGBlock_Temp_ini_degC
  Divide : Product  Inputs=/*
  Integrator : Integrator
  degC->K : Subsystem
  T_ENGBlock3_K : Outport
  T_ENGBlock2_K : Outport  Port=2
  T_ENGBlock1_K : Outport  Port=3
  wires:
  PHI_ENGBlock2_W/1 -> Add/3
  PHI_ENGBlock1_W/1 -> Add/1
  Constant/1 -> Divide/1
  Add/1 -> Divide/2
  Divide/1 -> Integrator/1
  Integrator/1 -> Add1/2
  Add1/1 -> T_ENGBlock2_K/1, T_ENGBlock1_K/1, T_ENGBlock3_K/1
  PHI_ENGBlock3_W/1 -> Add/2
  Constant1/1 -> degC->K/1(degC)
  degC->K/1(K) -> Add1/1

== system METI_TRAMI_Thermal_ver01_Jmaab_2018b_Intg/Vehicle/PTTH/ENGTH_PNT/ENGTH/ENGOil2Coolant_Heat_Resistance ==
  T_ENGOil_Resi2_K : Inport
  T_Coolant_Resi3_K : Inport  Port=2
  Add : Sum  Inputs=+-
  Constant : Constant  Value=ENG_PNT_ENGOil2Coolant_Heat_Resi_KpW
  Divide : Product  Inputs=*/
  Gain : Gain  Gain=-1
  Gain1 : Gain
  PHI_ENGOil_Resi2_W : Outport
  PHI_Coolant_Resi3_W : Outport  Port=2
  wires:
  T_ENGOil_Resi2_K/1 -> Add/1
  T_Coolant_Resi3_K/1 -> Add/2
  Constant/1 -> Divide/2
  Add/1 -> Divide/1
  Divide/1 -> Gain/1, Gain1/1
  Gain/1 -> PHI_ENGOil_Resi2_W/1
  Gain1/1 -> PHI_Coolant_Resi3_W/1

== system METI_TRAMI_Thermal_ver01_Jmaab_2018b_Intg/Vehicle/PTTH/ENGTH_PNT/ENGTH/ENGOil_Heat_Capacity ==
  PHI_ENGOil2_W : Inport
  PHI_ENGOil1_W : Inport  Port=2
  Add : Sum
  Add1 : Sum
  Constant : Constant  Value=ENG_PNT_ENGOil_Heat_Capa_JpK
  Constant1 : Constant  Value=ENG_PNT_ENGOil_Temp_ini_degC
  Divide : Product  Inputs=/*
  Integrator : Integrator
  degC->K : Subsystem
  T_ENGOil2_K : Outport
  T_ENGOil1_K : Outport  Port=2
  wires:
  PHI_ENGOil2_W/1 -> Add/2
  PHI_ENGOil1_W/1 -> Add/1
  Constant/1 -> Divide/1
  Add/1 -> Divide/2
  Divide/1 -> Integrator/1
  Integrator/1 -> Add1/2
  Add1/1 -> T_ENGOil2_K/1, T_ENGOil1_K/1
  Constant1/1 -> degC->K/1(degC)
  degC->K/1(K) -> Add1/1

== system METI_TRAMI_Thermal_ver01_Jmaab_2018b_Intg/Vehicle/PTTH/ENGTH_PNT/ENGTH/ENGOil_Heat_Capacity1 ==
  PHI_Cylinder_Head1_W : Inport
  PHI_Cylinder_Head2_W : Inport  Port=2
  Add : Sum
  Add1 : Sum
  Constant : Constant  Value=ENG_PNT_Cylinder_Head_Heat_Capa_JpK
  Constant1 : Constant  Value=ENG_PNT_Cylinder_Head_Temp_ini_degC
  Divide : Product  Inputs=/*
  Integrator : Integrator
  degC->K : Subsystem
  T_Cylinder_Head1_K : Outport
  T_Cylinder_Head2_K : Outport  Port=2
  wires:
  PHI_Cylinder_Head2_W/1 -> Add/2
  PHI_Cylinder_Head1_W/1 -> Add/1
  Constant/1 -> Divide/1
  Add/1 -> Divide/2
  Divide/1 -> Integrator/1
  Integrator/1 -> Add1/2
  Add1/1 -> T_Cylinder_Head2_K/1, T_Cylinder_Head1_K/1
  Constant1/1 -> degC->K/1(degC)
  degC->K/1(K) -> Add1/1

== system METI_TRAMI_Thermal_ver01_Jmaab_2018b_Intg/Vehicle/PTTH/ENGTH_PNT/ENGTH/Water_Pump ==
  ENG_PNT_Voltage_WP_V : Inport
  1-D Lookup Table : Lookup_n-D  NumberOfTableDimensions=1  BreakpointsForDimension1=ENG_PNT_Qv_Water_Pump_x_V_WP  Table=ENG_PNT_Qv_Water_Pump_m3ps  InternalRulePriority=Speed  RndMeth=Simplest  InputSameDT=on
  Qv_Coolant_m3ps : Outport
  wires:
  ENG_PNT_Voltage_WP_V/1 -> 1-D Lookup Table/1
  1-D Lookup Table/1 -> Qv_Coolant_m3ps/1

== system METI_TRAMI_Thermal_ver01_Jmaab_2018b_Intg/Vehicle/PTTH/RDTH_PNT/RDTH/ENGBlock2Coolant_Heat_Resistance ==
  T_RDCoolant_Resi1_K : Inport
  T_Thermostat_Resi1_K : Inport  Port=2
  1-D Lookup Table : Lookup_n-D  NumberOfTableDimensions=1  BreakpointsForDimension1=RD_PNT_Thermostat_Heat_Resi_KpW_T_Coolant  Table=RD_PNT_Thermostat_Heat_Resi_KpW  InternalRulePriority=Speed  RndMeth=Simplest  InputSameDT=on
  Add : Sum  Inputs=+-
  Divide : Product  Inputs=*/
  Gain : Gain  Gain=-1
  Gain1 : Gain
  K->degC : Subsystem
  PHI_RDCoolant_Resi1_W : Outport
  PHI_Thermostat_Resi1_W : Outport  Port=2
  tag scope: RD_PNT_Thermostat_Heat_Resi_KpW=global
  wires:
  Add/1 -> Divide/1
  Divide/1 -> Gain/1, Gain1/1
  Gain/1 -> PHI_Thermostat_Resi1_W/1
  T_Thermostat_Resi1_K/1 -> Add/1, K->degC/1(K)
  T_RDCoolant_Resi1_K/1 -> Add/2
  Gain1/1 -> PHI_RDCoolant_Resi1_W/1
  K->degC/1(degC) -> 1-D Lookup Table/1
  1-D Lookup Table/1 -> [RD_PNT_Thermostat_Heat_Resi_KpW], Divide/2

== system METI_TRAMI_Thermal_ver01_Jmaab_2018b_Intg/Vehicle/PTTH/RDTH_PNT/RDTH/RDCoolant2Air_Heat_Resistance ==
  T_RD_Air_Resi_K : Inport
  "RD_PNT_RDCore_Heat_Resi_KpW " : Inport  Port=2
  T_RDCoolant_Resi2_K : Inport  Port=3
  Add : Sum  Inputs=+-
  Divide : Product  Inputs=*/
  Gain : Gain  Gain=-1
  Gain1 : Gain
  PHI_RD_Air_Resi1_W : Outport
  PHI_RDCoolant_Resi2_W : Outport  Port=2
  wires:
  "RD_PNT_RDCore_Heat_Resi_KpW "/1 -> Divide/2
  Add/1 -> Divide/1
  Divide/1 -> Gain/1, Gain1/1
  Gain/1 -> PHI_RDCoolant_Resi2_W/1
  T_RDCoolant_Resi2_K/1 -> Add/1
  T_RD_Air_Resi_K/1 -> Add/2
  Gain1/1 -> PHI_RD_Air_Resi1_W/1

== system METI_TRAMI_Thermal_ver01_Jmaab_2018b_Intg/Vehicle/PTTH/RDTH_PNT/RDTH/RDCoolant_Heat_Capacity ==
  PHI_RDCoolant1_W : Inport
  PHI_RDCoolant2_W : Inport  Port=2
  Add : Sum
  Add1 : Sum
  Constant : Constant  Value=RD_PNT_RDCoolant_Heat_Capa_JpK
  Constant1 : Constant  Value=RD_PNT_RDCoolant_Temp_ini_degC
  Divide : Product  Inputs=/*
  Integrator : Integrator
  degC->K : Subsystem
  T_RDCoolant1_K : Outport
  T_RDCoolant2_K : Outport  Port=2
  wires:
  PHI_RDCoolant2_W/1 -> Add/2
  PHI_RDCoolant1_W/1 -> Add/1
  Constant/1 -> Divide/1
  Add/1 -> Divide/2
  Divide/1 -> Integrator/1
  Integrator/1 -> Add1/2
  Add1/1 -> T_RDCoolant2_K/1, T_RDCoolant1_K/1
  Constant1/1 -> degC->K/1(degC)
  degC->K/1(K) -> Add1/1

== system METI_TRAMI_Thermal_ver01_Jmaab_2018b_Intg/Vehicle/PTTH/RDTH_PNT/RDTH/RD_Core_Heat_Resi_Calc ==
  note: ラジエターファンの動作で
      | 発生する風速
  note: 車両の走行によって
      | ラジエターグリルに発生する風速
  note: ラジエターファンの動作で
      | ラジエターコアに当たる風量
  note: 車両の走行によって
      | ラジエターコアに当たる風量
  RD_PNT_Voltage_RDFan_V : Inport
  v_VL_PNT_kmph : Inport  Port=2
  1-D Lookup Table : Lookup_n-D  NumberOfTableDimensions=1  BreakpointsForDimension1=RD_PNT_RDCore_Heat_Resi_KpW_x_Wind_m3ps  Table=RD_PNT_RDCore_Heat_Resi_KpW  InternalRulePriority=Speed  RndMeth=Simplest  InputSameDT=on
  1-D Lookup Table1 : Lookup_n-D  NumberOfTableDimensions=1  BreakpointsForDimension1=RD_PNT_v_RDFan_Wind_vel_mps_x_V_RDFan  Table=RD_PNT_v_RDFan_Wind_vel_mps  InternalRulePriority=Speed  RndMeth=Simplest  InputSameDT=on
  Abs : Abs
  Add : Sum
  Constant : Constant  Value=RD_PNT_RDFan_area_m2
  Constant1 : Constant  Value=RD_PNT_RDGrill_area_m2
  Product : Product
  Product1 : Product
  gain1 : Gain  Gain=kmph2mps
  "RD_PNT_RDCore_Heat_Resi_KpW " : Outport
  wires:
  RD_PNT_Voltage_RDFan_V/1 -> 1-D Lookup Table1/1
  Constant/1 -> Product/2
  v_VL_PNT_kmph/1 -> gain1/1
  Constant1/1 -> Product1/2
  Product/1 -> Add/1
  Product1/1 -> Add/2
  Add/1 -> Abs/1
  1-D Lookup Table/1 -> "RD_PNT_RDCore_Heat_Resi_KpW "/1
  Abs/1 -> 1-D Lookup Table/1
  1-D Lookup Table1/1 -> Product/1
  gain1/1 -> Product1/1

== system METI_TRAMI_Thermal_ver01_Jmaab_2018b_Intg/Vehicle/TM_PNT/TM_PNT/TM_PNT/DF_PNT ==
  note: DF効率
  note: 車両を動かす側が正
  w_DF_PNT_DN_radps : Inport
  w_DF_PNT_UP_radps : Inport  Port=2
  T_DF_PNT_K : Inport  Port=3
  Constant4 : Constant  Value=DF_PNT_DF_gear
  DriveShaft : Subsystem
  Product4 : Product  Inputs=*/  RndMeth=Zero
  Product7 : Product  Inputs=*/  RndMeth=Zero
  Q_cal1 : METI_Lib_vehicle_model/P_cal  Type_energy=回転運動  Type_output_energy=出力  Power_name=Po_  t_Workspace_Name=DF_PNT_MECK  P_VariableName=Po_DF_PNT_MECK  Across_VariableName=w_DF_PNT_MECK  Throgh_VariableName=tq_DF_PNT_MECK
  Q_cal4 : METI_Lib_vehicle_model/P_cal  Type_energy=回転運動  Type_output_energy=損失  Power_name=Pl_  t_Workspace_Name=DF_PNT_MECK_LOSS  P_VariableName=Pl_DF_PNT_MECK_LOSS  Across_VariableName=w_DF_PNT_MECK_LOSS  Throgh_VariableName=tq_DF_PNT_MECK_LOSS
  Terminator : Terminator
  Terminator3 : Terminator
  eta_DF : Constant  Value=DF_PNT_eta_DF
  eta_cal : METI_Lib_vehicle_model/eta_cal  SystemSampleTime=-1
  trq_DS_PNT_Nm : Outport
  trq_DFNT_Nm : Outport  Port=2
  PHI_DF_PNT_W : Outport  Port=3
  wires:
  w_DF_PNT_UP_radps/1 -> Product4/1, Q_cal4/1, Q_cal1/1
  eta_DF/1 -> eta_cal/1
  eta_cal/2 -> Q_cal1/2, trq_DFNT_Nm/1  "trq_DFNT_Nm"
  eta_cal/1 -> Q_cal4/2
  Q_cal1/1 -> Terminator3/1
  Constant4/1 -> Product7/2, Product4/2
  Product7/1 -> eta_cal/2
  DriveShaft/1(trq_DS_PNT_in_Nm) -> trq_DS_PNT_Nm/1  "trq_DS_PNT_Nm"
  Product4/1 -> DriveShaft/2(w_DS_PNT_in_radps)
  w_DF_PNT_DN_radps/1 -> DriveShaft/1(w_TR_PNT_radps)
  DriveShaft/2(trq_DF_PNT_Nm) -> Product7/1
  Q_cal4/1 -> PHI_DF_PNT_W/1
  T_DF_PNT_K/1 -> Terminator/1

== system METI_TRAMI_Thermal_ver01_Jmaab_2018b_Intg/Vehicle/TM_PNT/TM_PNT/TM_PNT/K->degC ==
  K : Inport
  Constant2 : Constant  Value=K2degC
  Sum : Sum  Inputs=++|
  degC : Outport
  wires:
  K/1 -> Sum/2
  Constant2/1 -> Sum/1
  Sum/1 -> degC/1

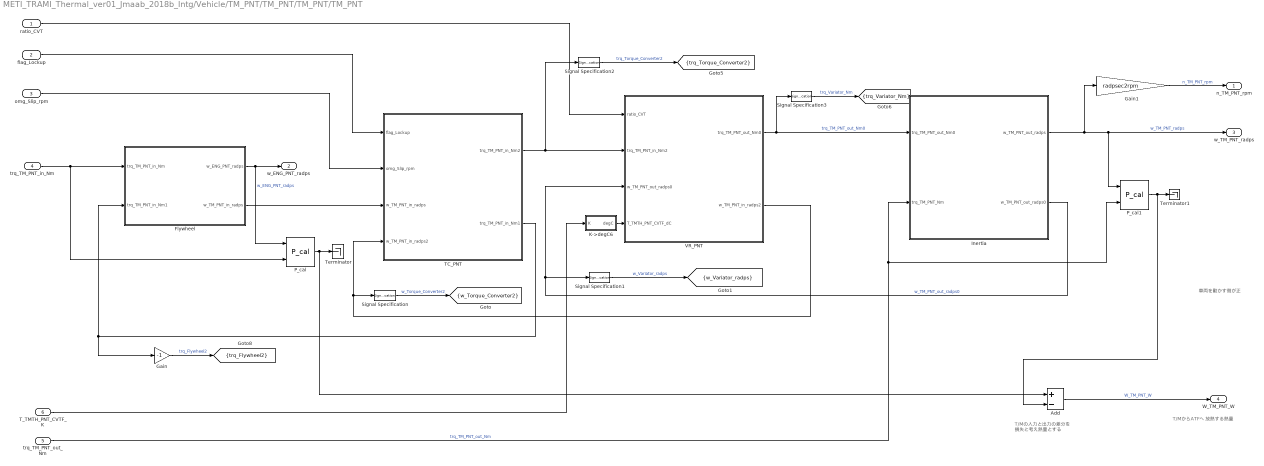
== system METI_TRAMI_Thermal_ver01_Jmaab_2018b_Intg/Vehicle/TM_PNT/TM_PNT/TM_PNT/TM_PNT ==
  note: 車両を動かす側が正
  note: T/MからATFへ
      | 放熱する熱量
  note: T/Mの入力と出力の差分を
      | 損失と考え熱量とする
  ratio_CVT : Inport
  flag_Lockup : Inport  Port=2
  omg_Slip_rpm : Inport  Port=3
  trq_TM_PNT_in_Nm : Inport  Port=4
  trq_TM_PNT_out_Nm : Inport  Port=5
  T_TMTH_PNT_CVTF_K : Inport  Port=6
  Add : Sum  Inputs=+-
  Flywheel : Subsystem
  Gain : Gain  Gain=-1
  Gain1 : Gain  Gain=radpsec2rpm
  Inertia : Subsystem
  K->degC6 : Subsystem
  P_cal : METI_Lib_vehicle_model/P_cal  Type_energy=回転運動  Type_output_energy=出力  Power_name=Po_  t_Workspace_Name=TM_PNT_MECK_UP  P_VariableName=Po_TM_PNT_MECK_UP  Across_VariableName=w_TM_PNT_MECK_UP  Throgh_VariableName=tq_TM_PNT_MECK_UP
  P_cal1 : METI_Lib_vehicle_model/P_cal  Type_energy=回転運動  Type_output_energy=出力  Power_name=Po_  t_Workspace_Name=TM_PNT_MECK_DN  P_VariableName=Po_TM_PNT_MECK_DN  Across_VariableName=w_TM_PNT_MECK_DN  Throgh_VariableName=tq_TM_PNT_MECK_DN
  Signal Specification{,1..3} (4 alike) : SignalSpecification
  TC_PNT : Subsystem
  Terminator : Terminator
  Terminator1 : Terminator
  VR_PNT : Subsystem
  n_TM_PNT_rpm : Outport
  w_ENG_PNT_radps : Outport  Port=2
  w_TM_PNT_radps : Outport  Port=3
  W_TM_PNT_W : Outport  Port=4
  tag scope: trq_Flywheel2=scoped, trq_Torque_Converter2=scoped, trq_Variator_Nm=scoped, w_Torque_Converter2=scoped, w_Variator_radps=scoped
  wires:
  VR_PNT/2(w_TM_PNT_in_radps2) -> Signal Specification/1, TC_PNT/4(w_TM_PNT_in_radps2)
  TC_PNT/1(trq_TM_PNT_in_Nm2) -> Signal Specification2/1, VR_PNT/2(trq_TM_PNT_in_Nm2)
  flag_Lockup/1 -> TC_PNT/1(flag_Lockup)
  omg_Slip_rpm/1 -> TC_PNT/2(omg_Slip_rpm)
  ratio_CVT/1 -> VR_PNT/1(ratio_CVT)
  TC_PNT/2(trq_TM_PNT_in_Nm1) -> Gain/1, Flywheel/2(trq_TM_PNT_in_Nm1)
  Flywheel/2(w_TM_PNT_in_radps) -> TC_PNT/3(w_TM_PNT_in_radps)
  Flywheel/1(w_ENG_PNT_radps) -> w_ENG_PNT_radps/1, P_cal/1  "w_ENG_PNT_radps"
  trq_TM_PNT_in_Nm/1 -> P_cal/2, Flywheel/1(trq_TM_PNT_in_Nm)
  Inertia/1(w_TM_PNT_out_radps) -> w_TM_PNT_radps/1, P_cal1/1, Gain1/1  "w_TM_PNT_radps"
  Gain1/1 -> n_TM_PNT_rpm/1  "n_TM_PNT_rpm"
  P_cal/1 -> Add/1, Terminator/1
  P_cal1/1 -> Terminator1/1, Add/2
  trq_TM_PNT_out_Nm/1 -> Inertia/2(trq_TM_PNT_Nm), P_cal1/2  "trq_TM_PNT_out_Nm"
  Inertia/2(w_TM_PNT_out_radps0) -> Signal Specification1/1, VR_PNT/3(w_TM_PNT_out_radps0)  "w_TM_PNT_out_radps0"
  VR_PNT/1(trq_TM_PNT_out_Nm0) -> Signal Specification3/1, Inertia/1(trq_TM_PNT_out_Nm0)  "trq_TM_PNT_out_Nm0"
  Add/1 -> W_TM_PNT_W/1  "W_TM_PNT_W"
  T_TMTH_PNT_CVTF_K/1 -> K->degC6/1(K)
  Gain/1 -> [trq_Flywheel2]  "trq_Flywheel2"
  K->degC6/1(degC) -> VR_PNT/4(T_TMTH_PNT_CVTF_dC)
  Signal Specification/1 -> [w_Torque_Converter2]  "w_Torque_Converter2"
  Signal Specification1/1 -> [w_Variator_radps]  "w_Variator_radps"
  Signal Specification2/1 -> [trq_Torque_Converter2]  "trq_Torque_Converter2"
  Signal Specification3/1 -> [trq_Variator_Nm]  "trq_Variator_Nm"

== system METI_TRAMI_Thermal_ver01_Jmaab_2018b_Intg/Driver/Driver/Driver/Caliculate_Opeining_Accel/FB/Filter ==
  In1 : Inport
  Gain3 : Gain  Gain=10
  Gain4 : Gain  Gain=0.1
  Rounding Function : Rounding  Operator=round
  Out1 : Outport
  wires:
  Rounding Function/1 -> Gain4/1
  In1/1 -> Gain3/1
  Gain3/1 -> Rounding Function/1
  Gain4/1 -> Out1/1

== system METI_TRAMI_Thermal_ver01_Jmaab_2018b_Intg/Driver/Driver/Driver/Caliculate_Opeining_Accel/FF/Air_Resistance ==
  V_tgt : Inport
  V_wind : Constant  Value=VL_PNT_V_wind
  cal_Air_resi1 : METI_Lib_vehicle_model/vehicle_model/cal_Air_resi  Vel_max=200
  F_air_resi : Outport
  wires:
  V_tgt/1 -> cal_Air_resi1/1
  V_wind/1 -> cal_Air_resi1/2
  cal_Air_resi1/1 -> F_air_resi/1

== system METI_TRAMI_Thermal_ver01_Jmaab_2018b_Intg/Driver/Driver/Driver/Caliculate_Opeining_Accel/FF/Cal_M_ENG_jiku2 ==
  note: 軸トルクマップ
  FF_trq_accel_Nm : Inport
  pre_n_eng_rpm : Inport  Port=2
  2-D Lookup Table : Lookup_n-D  BreakpointsForDimension1=ENG_trq_rev  BreakpointsForDimension2=ENG_rpm  Table=ENG_throttle_rev  ExtrapMethod=Clip  UseLastTableValue=on  RndMeth=Simplest  InputSameDT=on
  2-D Lookup Table1 : Lookup_n-D  BreakpointsForDimension1=ENG_PNT_trq_Nm_map_y_throttle  BreakpointsForDimension2=ENG_PNT_trq_Nm_map_x_rpm  Table=ENG_PNT_trq_Nm_map  ExtrapMethod=Clip  UseLastTableValue=on  RndMeth=Simplest  InputSameDT=on
  Constant : Constant  Value=0
  Subsystem : Subsystem
  Sum : Sum  Inputs=|++
  FF_open_accel_per : Outport
  wires:
  FF_trq_accel_Nm/1 -> Sum/1
  2-D Lookup Table/1 -> Subsystem/1(In1)
  pre_n_eng_rpm/1 -> 2-D Lookup Table/2, 2-D Lookup Table1/2
  Constant/1 -> 2-D Lookup Table1/1
  Sum/1 -> 2-D Lookup Table/1
  2-D Lookup Table1/1 -> Sum/2
  Subsystem/1(Out1) -> FF_open_accel_per/1

== system METI_TRAMI_Thermal_ver01_Jmaab_2018b_Intg/Driver/Driver/Driver/Caliculate_Opeining_Accel/FF/Inertial_Resistance ==
  V_tgt : Inport
  Constant : Constant  Value=M
  Derivative : Derivative
  Divide : Product  OutDataTypeStr=Inherit: Same as first input
  F_Inertia : Outport
  wires:
  Constant/1 -> Divide/2
  Derivative/1 -> Divide/1
  Divide/1 -> F_Inertia/1
  V_tgt/1 -> Derivative/1

== system METI_TRAMI_Thermal_ver01_Jmaab_2018b_Intg/Driver/Driver/Driver/Caliculate_Opeining_Accel/FF/Rolling_Resistance ==
  note: 20151211修正
      |
      | 空気抵抗と表現を統一する、ため
      | -1のGainを削除
  V_tgt : Inport
  cal_roll_resi1 : METI_Lib_vehicle_model/vehicle_model/cal_roll_resi  Myu_tire=myu  Vehicle_Mass=M  Gravi_acc=g
  F_rollresi : Outport
  wires:
  V_tgt/1 -> cal_roll_resi1/1
  cal_roll_resi1/1 -> F_rollresi/1

== system METI_TRAMI_Thermal_ver01_Jmaab_2018b_Intg/Driver/Driver_TRAMI/Driver2/Caliculate_Opeining_Accel/FB/Filter ==
  In1 : Inport
  Gain3 : Gain  Gain=10
  Gain4 : Gain  Gain=0.1
  Rounding Function : Rounding  Operator=round
  Out1 : Outport
  wires:
  Rounding Function/1 -> Gain4/1
  In1/1 -> Gain3/1
  Gain3/1 -> Rounding Function/1
  Gain4/1 -> Out1/1

== system METI_TRAMI_Thermal_ver01_Jmaab_2018b_Intg/Driver/Driver_TRAMI/Driver2/Caliculate_Opeining_Accel/FF/Air_Resistance ==
  V_tgt : Inport
  V_wind : Constant  Value=VL_PNT_V_wind
  cal_Air_resi1 : METI_Lib_vehicle_model/vehicle_model/cal_Air_resi  Vel_max=200
      settings: SourceProductName=The database C:\Users\k-uekata\AppData\Roaming\MathWorks\MATLAB\R2018b\slblocks_master.db is locked, or a table in the database is locked. (database is locked)
  F_air_resi : Outport
  wires:
  V_tgt/1 -> cal_Air_resi1/1
  V_wind/1 -> cal_Air_resi1/2
  cal_Air_resi1/1 -> F_air_resi/1
